simulink model "QD2_IOCheck_2021b"  (R2021b)
settings: Solver=ode2  StartTime=0.0  StopTime=inf  FixedStep=1/1000  RelTol=1e-3  EnableMultiTasking=on
InitFcn:
  | Motor_Mapping_7_Inch
undefined symbols (not defined in the file): datetime, HIL, KT, log_QD2_, m, Motor_Matrix, qc_get_step_size, saved_data
libraries: quarc_library x44, simulink x6, simulink_extras x1
(part 1 of 2)
settings Model: DataTypeOverride=Double  MinMaxOverflowLogging=ForceOff  SimulationMode=external  ExtModeTrigElement=1  ExtModeTrigDuration=10000  ExtModeTrigLevel=0.400000  Creator=dmadill  LastModifiedBy=jpineros
settings SolverCC: AlgebraicLoopSolver=TrustRegion  PositivePriorityOrder=on  AutoInsertRateTranBlk=on
settings DataIOCC: ReturnWorkspaceOutputs=off
settings DebuggingCC: ArithmeticOperatorsInVariantConditions=warning
settings HardwareCC: ProdBitPerLong=64  ProdLargestAtomicInteger=LongLong  ProdLargestAtomicFloat=Double  ProdLongLongMode=on  ProdHWDeviceType=ARM Compatible->ARM 64-bit (LP64)
settings SFSimCC: SimUseLocalCustomCode=off  CustomCodeUndefinedFunction=UseInterfaceOnly
settings RTWCC: Description=QUARC Linux QDrone2 Target Using Toolchain  SystemTargetFile=quarc_linux_qdrone2.tlc  RTWUseLocalCustomCode=off  Toolchain=QUARC linux_qdrone2 | gmake (64-bit Windows)  BuildConfiguration=Faster Runs
settings CodeAppCC: StateflowObjectComments=on
settings STFCustomTargetCC: ConcurrentExecutionCompliant=on  UseToolchainInfoCompliant=on  SystemTargetFile=quarc_linux_qdrone2.tlc
settings GRTTargetCC: TargetLangStandard=C89/C90 (ANSI)  ParMdlRefBuildCompliant=off  CompOptLevelCompliant=off  CombineOutputUpdateFcns=off  MatFileLogging=off  CPPClassGenCompliant=off  GRTInterface=on  ExtMode=on  ExtModeMexFile=quarc_comm  ExtModeMexArgs='-w -d /tmp -uri %u','tcpip://192.168.55.1:17001'
settings ConfigComp: CovMetricSettings=dswe

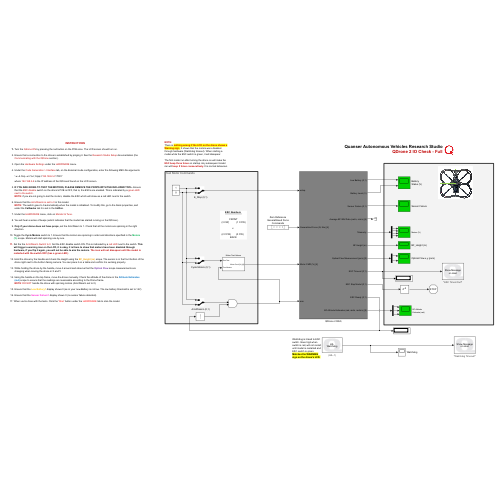
[thumbnail: Simulink's stored preview of the top-level diagram]
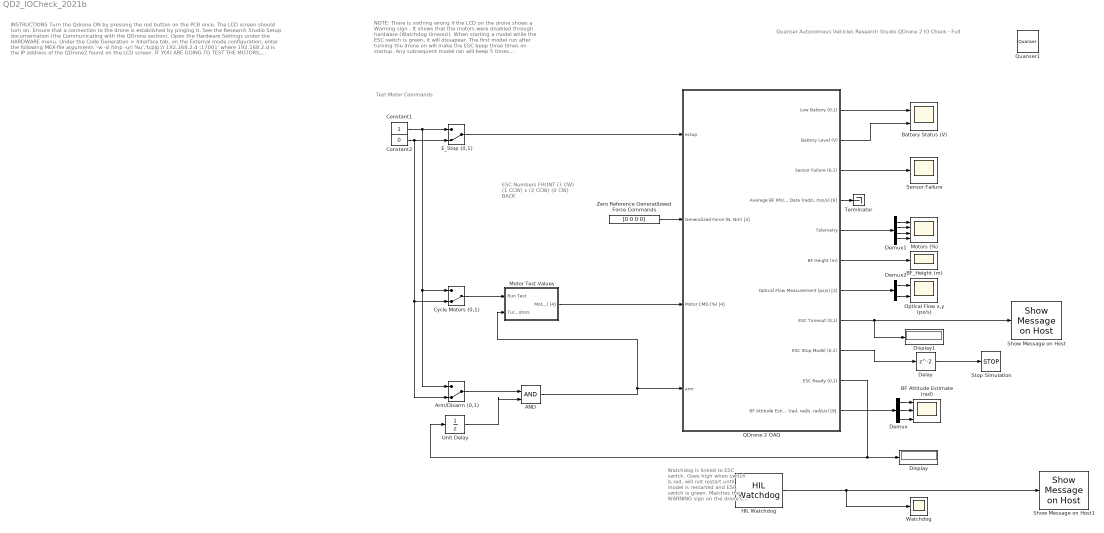
== system QD2_IOCheck_2021b ==
  note: Watchdog is linked to ESC switch. Goes high when switch is red, will not restart until model is restarted and ESC switch is green.
      | Matches the WARNING sign on the drone's LCD.
  note: Test Motor Commands
  note: Quanser Autonomous Vehicles Research Studio
      | QDrone 2 IO Check - Full
  note: ESC Numbers
      |
      | FRONT
      | (3 CW) (1 CCW)
      |
      | x
      |
      | (2 CCW) (0 CW)
      | BACK
  note: INSTRUCTIONS
      |
      | Turn the Qdrone ON by pressing the red button on the PCB once. The LCD screen should turn on.
      |
      | Ensure that a connection to the drone is established by pinging it. See the Research Studio Setup documentation (the Communicating with the QDrone section).
      |
      | Open the Hardware Settings under the HARDWARE menu.
      |
      | Under the Code Generation > Interface tab, on the External mode configuration, enter the following MEX-file arguments
      |
      | '-w -d /tmp -uri %u','tcpip:// 192.168.2.d :17001'
      |
      | where 192.168.2.d is the IP address of the QDrone2 found on the LCD screen.
      |
      | IF YOU ARE GOING TO TEST THE MOTORS, PLEASE REMOVE THE PROPS WITH THE INCLUDED TOOL. Ensure that the ESC disable switch on the drone's PCB is OFF, that is, the ESCs are enabled. This is indicated by a green LED next to the switch .
      | NOTE: if you are not going to test the motors, disable the ESC which will show as a red LED next to the switch.
      |
      | Ensure that the Arm/Disarm is set to 0 in this model.
      | NOTE: The switch goes to 0 automatically when the model is initialized. To modify this, go to the block properties, and under the Callbacks tab it is set in the InitFcn .
      |
      | Under the HARDWARE menu, click on Monitor & Tune .
      |
      | You will hear a series of beeps (which indicates that the model has started running on the QDrone).
      |
      | Only if your drone does not have props, set the Arm/Disarn to 1. Check that all the motors are spinning in the right direction.
      |
      | Toggle the Cycle Motors switch to 1. Ensure that the motors are spinning in order and directions specified in the Motors (%) scope. Motors will start spinning one by one.
      |
      | Set the the Arm/Disarm Switch to 0. Set the ESC disable switch ON. This is indicated by a red LED next to the switch. This will trigger a warning icon on the LCD, it is okay, it is there to show that motors have been disabled through hardware, if you flip it again, you will not be able to arm the motors. The icon will not dissapear until the model is restarted with the switch OFF (has a green LED.)
      |
      | Hold the drone by the handle and check the Height using the BF_Height (m) scope. The sensor is in the front bottom of the drone right next to the bottom facing camera. You can place it on a table and confirm it is working properly.
      |
      | While holding the drone by the handle, move it around and observe that the Optical Flow scope measurements are changing when moving the drone in X and Y.
      |
      | Using the handle on the top frame, move the drone manually. Check the attitude of the drone in the Attitude Estimates (rad) scope to ensure that the readings are reasonable according to the Drone frame.
      | NOTE : DO NOT handle the drone with spinning motors (Arm/Disarm set to 0).
      |
      | Ensure that the Low Battery? display shows 0 (as in your new Battery is not low. The low battery threshold is set to 14V)
      |
      | Ensure that the Sensor Failure? display shows 0 (no sensor failure detected).
      |
      | When you're done with the tests, Click the ' Stop ' button under the HARDWARE tab to stop the model.
  note: NOTE:
      | There is nothing wrong if the LCD on the drone shows a Warning sign . It shows that the motors were disabled through hardware (Watchdog timeout). When starting a model while the ESC switch is green, it will dissapear.
      |
      | The first model run after turning the drone on will make the ESC beep three times on startup. Any subsequent model ran will beep 5 times consecutively. It is normal behaviour.
  AND : Logic  IconShape=distinctive  AllPortsSameDT=off  OutDataTypeStr=boolean
  Arm/Disarm (0,1) : ManualSwitch  InitFcn=set_param(gcb,'sw','0')  CurrentSetting=0
  "BF Attitude Estimate (rad) " : Scope  NumInputPorts=3
  BF_Height (m) : Scope
  Battery Status (V) : Scope  NumInputPorts=2
  Constant1 : Constant
  Constant2 : Constant  Value=0
  Cycle Motors (0,1) : ManualSwitch  InitFcn=set_param(gcb,'sw','0')  CurrentSetting=0
  Delay : Delay
  Demux : Demux  Outputs=3
  Demux1 : Demux
  Demux2 : Demux  Outputs=2
  Display : Display
  Display1 : Display
  E_Stop (0,1) : ManualSwitch  CurrentSetting=0
  HIL Watchdog : quarc_library/Data Acquisition/Generic/Watchdog/HIL Watchdog  object_name=HIL-1  timeout=0.1  sample_time=qc_get_step_size  active=off
      settings: AttributesFormatString=(%<object_name>)  SourceProductName=QUARC Targets
  Motor Test Values : Subsystem
  Motors (%) : Scope  NumInputPorts=4
  Optical Flow x,y (px/s) : Scope  NumInputPorts=2
  QDrone 2 DAQ : Subsystem
  Quanser1 : quarc_library/Logos/Quanser
  Sensor Failure : Scope
  Show Message on Host : quarc_library/Sinks/Error Handling/Show Message on Host  message_type=Fixed error message  message_icon=Error  message=ESC Timed Out!
      settings: AttributesFormatString="\"%<message>\""  SourceProductName=QUARC Targets
  Show Message on Host1 : quarc_library/Sinks/Error Handling/Show Message on Host  message_type=Fixed error message  message_icon=Error  message=Watchdog Timeout!
      settings: AttributesFormatString="\"%<message>\""  SourceProductName=QUARC Targets
  Stop Simulation : Stop
  Terminator : Terminator
  Unit Delay : UnitDelay  SampleTime=-1  HasFrameUpgradeWarning=on
  Watchdog : Scope
  Zero Reference Generatlizeed Force Commands : Constant  Value=[0 0 0 0]
  wires:
  Constant2/1 -> Arm/Disarm (0,1)/2, Cycle Motors (0,1)/2, E_Stop (0,1)/2
  Constant1/1 -> E_Stop (0,1)/1, Arm/Disarm (0,1)/1, Cycle Motors (0,1)/1
  Demux/1 -> "BF Attitude Estimate (rad) "/1
  Demux/2 -> "BF Attitude Estimate (rad) "/2
  Demux/3 -> "BF Attitude Estimate (rad) "/3
  Demux2/1 -> Optical Flow x,y (px/s)/1
  Demux2/2 -> Optical Flow x,y (px/s)/2
  Demux1/3 -> Motors (%)/3
  Demux1/2 -> Motors (%)/2
  Demux1/4 -> Motors (%)/4
  Demux1/1 -> Motors (%)/1
  HIL Watchdog/1 -> Show Message on Host1/1, Watchdog/1
  Cycle Motors (0,1)/1 -> Motor Test Values/1(Run Test)
  E_Stop (0,1)/1 -> QDrone 2 DAQ/1(estop)
  Motor Test Values/1(Motor Cmd (%) [4]) -> QDrone 2 DAQ/3(Motor CMD (%) [4])
  QDrone 2 DAQ/5(Telemetry) -> Demux1/1
  QDrone 2 DAQ/1(Low Battery (0,1)) -> Battery Status (V)/1
  QDrone 2 DAQ/2(Battery Level (V)) -> Battery Status (V)/2
  QDrone 2 DAQ/6(BF Height (m)) -> BF_Height (m)/1
  QDrone 2 DAQ/7(Optical Flow Measurement (px/s) [2]) -> Demux2/1
  QDrone 2 DAQ/4("Average BF IMU Data (rad/s, m/s/s) [6]") -> Terminator/1
  QDrone 2 DAQ/3(Sensor Failure (0,1)) -> Sensor Failure/1
  QDrone 2 DAQ/10(ESC Ready (0,1)) -> Unit Delay/1, Display/1
  AND/1 -> QDrone 2 DAQ/4(arm), Motor Test Values/2(Turn Motors)
  Arm/Disarm (0,1)/1 -> AND/1
  Unit Delay/1 -> AND/2
  QDrone 2 DAQ/9(ESC Stop Model (0,1)) -> Delay/1
  QDrone 2 DAQ/8(ESC Timeout (0,1)) -> Show Message on Host/1, Display1/1
  Delay/1 -> Stop Simulation/1
  QDrone 2 DAQ/11("BF Attitude Estimates (rad, rad/s, rad/s/s) [9]") -> Demux/1
  Zero Reference Generatlizeed Force Commands/1 -> QDrone 2 DAQ/2("Generalized Force (N, Nm) [4]")

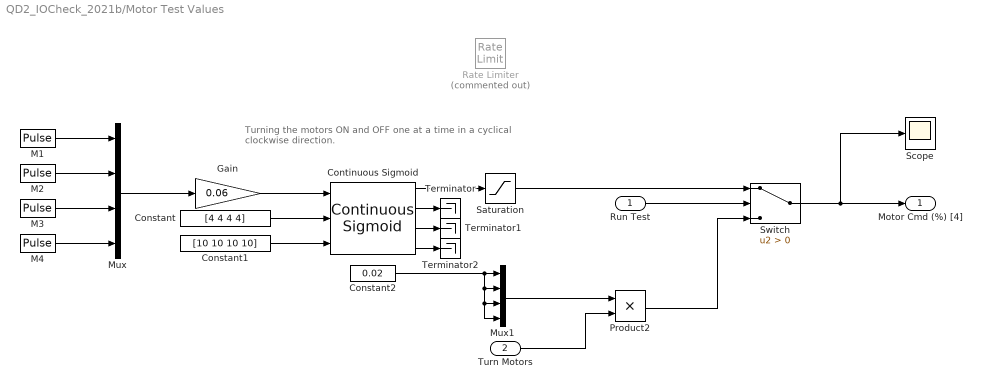
== system QD2_IOCheck_2021b/Motor Test Values ==
  note: Turning the motors ON and OFF one at a time in a cyclical
      | clockwise direction.
  Run Test : Inport
  Turn Motors : Inport  Port=2
  Constant : Constant  Value=[4 4 4 4]
  Constant1 : Constant  Value=[10 10 10 10]
  Constant2 : Constant  Value=0.02
  Continuous Sigmoid : quarc_library/Sources/Sigmoids/Continuous Sigmoid  params_source=External (input ports)  max_velocity=10  max_acceleration=10  initial_position=0  initial_velocity=0  hold_off=0.5  input_sample_time=-1  output_sample_time=qc_get_step_size
      settings: SourceProductName=QUARC Targets
  Gain : Gain  Gain=0.06
  M1 : DiscretePulseGenerator  PulseType=Time based  Period=8  PulseWidth=12.5
  M2 : DiscretePulseGenerator  PulseType=Time based  Period=8  PulseWidth=12.5  PhaseDelay=6
  M3 : DiscretePulseGenerator  PulseType=Time based  Period=8  PulseWidth=12.5  PhaseDelay=2
  M4 : DiscretePulseGenerator  PulseType=Time based  Period=8  PulseWidth=12.5  PhaseDelay=4
  Mux : Mux
  Mux1 : Mux
  Product2 : Product
  Rate Limiter : RateLimiter  Commented=on  RisingSlewLimit=0.1  FallingSlewLimit=-0.1  SampleTimeMode=inherited
  Saturation : Saturate  UpperLimit=0.1  LowerLimit=0.02
  Scope : Scope
  Switch : Switch  Criteria=u2 > Threshold
  Terminator : Terminator
  Terminator1 : Terminator
  Terminator2 : Terminator
  Motor Cmd (%) [4] : Outport  VectorParamsAs1DForOutWhenUnconnected=off
  wires:
  M2/1 -> Mux/2
  M3/1 -> Mux/3
  M4/1 -> Mux/4
  M1/1 -> Mux/1
  Continuous Sigmoid/1 -> Saturation/1
  Mux/1 -> Gain/1
  Gain/1 -> Continuous Sigmoid/1
  Constant/1 -> Continuous Sigmoid/2
  Constant1/1 -> Continuous Sigmoid/3
  Product2/1 -> Switch/3
  Saturation/1 -> Switch/1
  Turn Motors/1 -> Product2/2
  Switch/1 -> Motor Cmd (%) [4]/1, Scope/1
  Run Test/1 -> Switch/2
  Mux1/1 -> Product2/1
  Constant2/1 -> Mux1/2, Mux1/4, Mux1/3, Mux1/1
  Continuous Sigmoid/2 -> Terminator/1
  Continuous Sigmoid/3 -> Terminator1/1
  Continuous Sigmoid/4 -> Terminator2/1

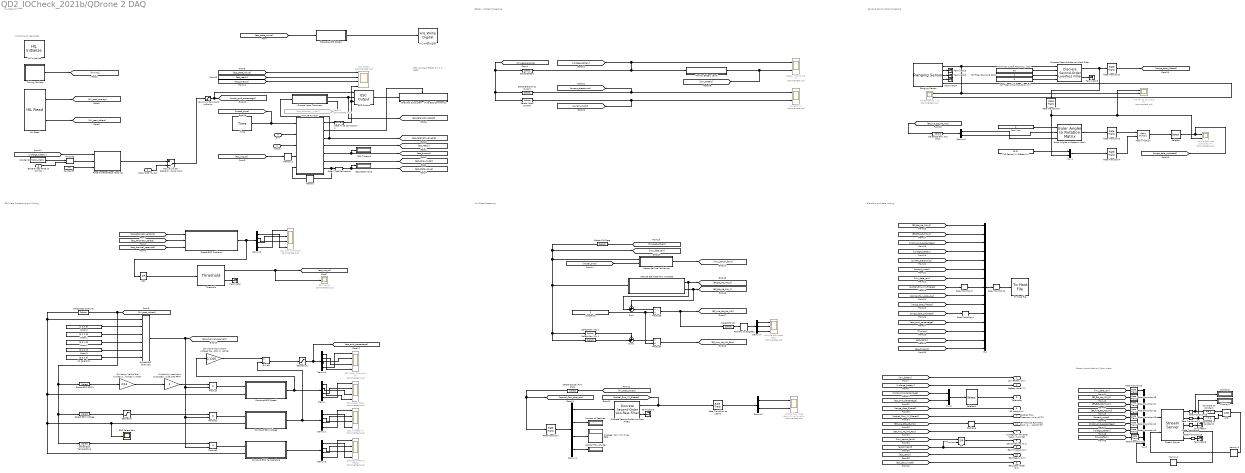
== system QD2_IOCheck_2021b/QDrone 2 DAQ ==
  note: Stream drone data to Python class
  note: HIL Read Write
  note: Blackbox and data routing
  note: ESC Numbers
      |
      | FRONT
      | 3 1
      |
      | 2 0
      | BACK
  note: Ranging Sensor Data Processing
  note: Initialize and read data
  note: ESC Data Processing and Writing
  note: IMU Data Processing
  note: Battery Voltage Processing
  estop : Inport
  "Generalized Force (N, Nm) [4]" : Inport  Port=2
  Motor CMD (%) [4] : Inport  Port=3
  arm : Inport  Port=4
  AND : Logic  IconShape=distinctive  AllPortsSameDT=off  OutDataTypeStr=boolean
  Attitude Estimate from IMU Data : Subsystem
  Attitude Estimates (deg) : Scope  Commented=on  NumInputPorts=3
  "Average, Max, Min Pixel Rate" : Display
  Battery Monitoring (V) : Scope  Commented=on  NumInputPorts=2
  Choose Motor Telemetry : Subsystem
  Compare To Constant : simulink/Logic and Bit Operations/Compare To Constant  relop===  const=2  OutDataTypeStr=boolean
  Compare To Constant1 : simulink/Logic and Bit Operations/Compare To Constant  relop=>=  const=0  OutDataTypeStr=boolean
  Constant1 : Constant  Value=2
  Constant2 : Constant  Value=Motor_Matrix  OutDataTypeStr=double
  Constant3 : Constant  Value=KT  OutDataTypeStr=double
  Construct ESC Speed : Subsystem
  Construct ESC Temperature : Subsystem
  Construct ESC Voltage : Subsystem
  Convert to equivalent voltage (based on motor Kv rating) : Gain  Gain=1/1300
  Currents (A) : Scope  Commented=on  NumInputPorts=2
  Data Type Conversion : DataTypeConversion  OutDataTypeStr=uint32
  Data Type Conversion1 : DataTypeConversion
  Demux{,1..3,8} (5 alike) : Demux
  Demux4 : Demux  Outputs=[2 1 3 1]
  Demux5 : Demux  Outputs=2
  Demux6 : Demux  Outputs=2
  Demux7 : Demux  Outputs=3
  Detect ESC Problems : Subsystem
  Discrete Second-Order Low-Pass Filter : quarc_library/Discrete/Discrete Second-Order Low-Pass Filter  params_source=External (input ports)  input_width=1  input_zeta=1  input_init=0  sample_time=qc_get_step_size*ceil(1/25/qc_get_step_size)
      settings: SourceProductName=QUARC Targets
  Discrete Second-Order Low-Pass Filter1 : quarc_library/Discrete/Discrete Second-Order Low-Pass Filter  params_source=Internal (dialog parameters)  input_width=1  input_zeta=1  input_init=0  sample_time=0.01
      settings: SourceProductName=QUARC Targets
  Display5 : Display
  Display6 : Display
  Divide : Product  Inputs=*/
  Divide by half of the number of poles in motor : Gain  Gain=2/14
  ESC Comm Problem : Scope  Commented=on  NumInputPorts=4
  ESC Motor Command (%) : Scope  Commented=on  NumInputPorts=4
  ESC Not OK : Scope  Commented=on
  ESC Output : quarc_library/Data Acquisition/Generic/Transformations/ESC Output  protocol=DShot (raw)
      settings: AttributesFormatString=%<protocol>  SourceProductName=QUARC Targets
  ESC Select Raw : Scope
  ESC Speed (RPM) : Scope  Commented=on  NumInputPorts=4
  ESC State Value : Display
  ESC States : Scope  Commented=on  NumInputPorts=4
  ESC Temperature (degC) : Scope  Commented=on  NumInputPorts=4
  ESC Timeout : Display
  ESC Voltage (V) : Scope  Commented=on  NumInputPorts=4
  Enabled Subsystem - Write ESC Commands : Subsystem  TreatAsAtomicUnit=on
  Euler Angles to Rotation Matrix : quarc_library/Math Operations/Matrices/Euler Angles to Rotation Matrix  menu_order=Relative Z-Y-X
      settings: SourceProductName=QUARC Targets
  Extract ESC Channels : MultiPortSwitch  DataPortOrder=Zero-based contiguous  Inputs=4  DataPortForDefault=Additional data port  zeroidx=on
  Force to percentage Mapping : MATLAB Function  TreatAsAtomicUnit=on
  Generate LED Pattern : Subsystem
  Goto19 : Goto  Commented=on  GotoTag=esc_telemetry_index
  HIL Initialize : quarc_library/Data Acquisition/Generic/Configuration/HIL Initialize  object_name=HIL-1  board_type=qdrone2  board_number=0  board_options=gyro0_fs=250;gyro0_rate=500;gyro0_bw=125;gyro0_ord=3;accel0_fs=16;accel0_rate=1000;accel0_bw=250;accel0_ord=3;temp0_bw=4000;gyro1_fs=250;gyro1_rate=500;gyro1_bw=125;gyro1_ord=3;accel1_fs=16;accel1_rate=1000;accel1_bw=400;accel1_ord=3;temp1_bw=4000;enc0_dir=0;enc1_dir=0;pwm03_dshot=1;opt_rate=121;  exclusive=off  active=on  hardware_clocks=[]  clock_modes=[]  initial_clock_frequencies=[]  set_clock_params_at_start=off  set_clock_params_at_switch_in=off  set_clock_frequencies_at_start=off  set_clock_frequencies_at_switch_in=off  analog_input_channels=[0:3]  analog_input_configurations=[]  analog_input_maximums=[3.3]  analog_input_minimums=[0]  set_analog_input_params_at_start=off  set_analog_input_params_at_switch_in=off  analog_output_channels=[]  analog_output_maximums=[]  analog_output_minimums=[]  initial_analog_outputs=[]  final_analog_outputs=[]  watchdog_analog_outputs=[]  set_analog_output_params_at_start=off  set_analog_output_params_at_switch_in=off  set_analog_outputs_at_start=off  set_analog_outputs_at_switch_in=off  set_analog_outputs_at_terminate=off  set_analog_outputs_at_switch_out=off  set_analog_outputs_on_watchdog=off  digital_input_channels=[0:5]  digital_output_channels=[6:11]  digital_output_configuration=[]  initial_digital_outputs=[0]  final_digital_outputs=[0]  watchdog_digital_outputs=[0 0 0 0 0 0]  set_digital_output_params_at_start=off  set_digital_output_params_at_switch_in=off  set_digital_outputs_at_start=on  set_digital_outputs_at_switch_in=off  set_digital_outputs_at_terminate=on  set_digital_outputs_at_switch_out=off  set_digital_outputs_on_watchdog=off  encoder_channels=[0:1]  quadrature=[4]  encoder_filter_frequency=100e6/1  initial_encoder_counts=[0]  set_encoder_params_at_start=on  set_encoder_params_at_switch_in=off  set_encoder_counts_at_start=on  set_encoder_counts_at_switch_in=off  pwm_channels=[0:5]  pwm_modes=[6 6 6 6 0]  pwm_frequency=[600000]  pwm_configuration=[0]  pwm_alignment=[0]  pwm_polarity=[1]  pwm_leading_deadband=[]  pwm_trailing_deadband=[]  initial_pwm_outputs=[0]  final_pwm_outputs=[0]  watchdog_pwm_outputs=[0]  set_pwm_params_at_start=on  set_pwm_params_at_switch_in=off  set_pwm_outputs_at_start=on  set_pwm_outputs_at_switch_in=off  set_pwm_outputs_at_terminate=on  set_pwm_outputs_at_switch_out=off  set_pwm_outputs_on_watchdog=on  other_output_channels=[]  initial_other_outputs=[]  final_other_outputs=[]  watchdog_other_outputs=[]  set_other_outputs_at_start=on  set_other_outputs_at_switch_in=off  set_other_outputs_at_terminate=on  set_other_outputs_at_switch_out=off  set_other_outputs_on_watchdog=off
  HIL Read : quarc_library/Data Acquisition/Generic/Immediate I//O/HIL Read  object_name=HIL-1  analog_channels=[3 1:2]  encoder_channels=[]  digital_channels=[]  other_channels=[3000:3002 4000:4002 3003:3005 4003:4005 17000:17006 17008:17009 17007 17010]  sample_time=qc_get_step_size  active=on  vector_output=on  data_type_mode=Inherit via back propagation  encoder_data_type=double  digital_data_type=boolean
  HIL Write Digital : quarc_library/Data Acquisition/Generic/Immediate I//O/HIL Write Digital  object_name=HIL-1  channels=[6:11]  sample_time=-1  active=off  vector_input=on
      settings: SourceProductName=QUARC Targets
  Height Estimate Compares (m) : Scope  Commented=on  NumInputPorts=2
  MATLAB Function : MATLAB Function  TreatAsAtomicUnit=on
  Manual Switch - Select Command Input : ManualSwitch  CurrentSetting=0
  Matrix Multiply : Product  Multiplication=Matrix(*)
  "Maximum Command Authority " : Saturate  UpperLimit=[1 1 1 1]  LowerLimit=[1 1 1 1]*0.025
  Memory : Memory
  Memory1 : Memory
  Memory2 : Memory  InheritSampleTime=on
  Memory3 : Memory  InheritSampleTime=on
  Monitor Battery Level : Subsystem
  Motor 0 : Constant  Value=[1 0 0 0]
  Motor 1 : Constant  Value=[0 1 0 0]
  Motor 2 : Constant  Value=[0 0 1 0]
  Motor 3 : Constant  Value=[0 0 0 1]
  Multiple by resolution (supposed to be 100 RPM) : Gain
  Mux : Mux  Inputs=15
  Mux1 : Mux  Inputs=2
  Mux2 : Mux  Inputs=2
  Mux3 : Mux  Inputs=9
  No selection : Constant  Value=[0 0 0 0]
  Number of Features : Display
  OR : Logic  Operator=OR  IconShape=distinctive  AllPortsSameDT=off  OutDataTypeStr=boolean
  OR1 : Logic  Operator=OR  Inputs=1  IconShape=distinctive  AllPortsSameDT=off  OutDataTypeStr=boolean
  Optical Flow Rate (Body Frame) (pixel/s) : Scope  Commented=on  NumInputPorts=2
  Optical Flow Shutter : Display
  Product : Product
  Product1 : Product
  Product2 : Product
  Product3 : Product  Inputs=*/
  Product4 : Product  Inputs=*/
  Product5 : Product  Multiplication=Matrix(*)
  Radians to Degrees : simulink_extras/Transformations/Radians to Degrees
  Ranging Sensor : quarc_library/Devices/Third-Party/Sensors/Ranging Sensor  sensor_type=VL53L1X Time-of-flight  uri=i2c-cpu://localhost:0?address='0x29',baud='400000',memsize='512'  ranging_distance=Long  timing_budget=0.033  measurement_period=0.040  output_mode=Fixed-size output  samples_per_revolution=1300  max_distance=0.050  max_angle=5  sample_time=qc_get_step_size*ceil(1/25/qc_get_step_size)  show_versions=off  active=on
      settings: SourceProductName=QUARC Targets
  Rate Transition : RateTransition  OutPortSampleTime=0.01
  Rate Transition to 100Hz : RateTransition  OutPortSampleTime=0.01
  Rate Transition{1..2,7..12,14..20} (15 alike) : RateTransition
  Rate Transition3 : RateTransition  OutPortSampleTime=qc_get_step_size*ceil(1/25/qc_get_step_size)
  Rate Transition4 : RateTransition  OutPortSampleTime=qc_get_step_size*ceil(1/25/qc_get_step_size)
  Rate Transition5 : RateTransition  OutPortSampleTime=qc_get_step_size*ceil(1/25/qc_get_step_size)
  Rate Transition6 : RateTransition  OutPortSampleTime=qc_get_step_size
  Reshape : Reshape
  Saturation : Saturate  UpperLimit=17  LowerLimit=10
  Saturation1 : Saturate  UpperLimit=1  LowerLimit=0
  Select Battery : Selector  InputPortWidth=3  IndexOptions=Index vector (dialog)  Indices=[1]  OutputSizes=1
  Select ESC Channel : Selector  InputPortWidth=23  IndexOptions=Index vector (dialog)  Indices=[22]  OutputSizes=1
  Select ESC RPPM : Selector  InputPortWidth=23  IndexOptions=Index vector (dialog)  Indices=[20]  OutputSizes=1
  Select ESC Temperature : Selector  InputPortWidth=23  IndexOptions=Index vector (dialog)  Indices=[23]  OutputSizes=1
  Select ESC Voltage : Selector  InputPortWidth=23  IndexOptions=Index vector (dialog)  Indices=[21]  OutputSizes=1
  Select Electronics Current : Selector  InputPortWidth=3  IndexOptions=Index vector (dialog)  Indices=[2]  OutputSizes=1
  Select Est Att : Selector  InputPortWidth=9  IndexOptions=Index vector (dialog)  Indices=[1:3]  OutputSizes=1
  Select Est Roll and Pitch : Selector  InputPortWidth=9  IndexOptions=Index vector (dialog)  Indices=[1:2]  OutputSizes=1
  Select IMU Data : Selector  InputPortWidth=23  IndexOptions=Index vector (dialog)  Indices=[1:12]  OutputSizes=1
  Select Motor Current : Selector  InputPortWidth=3  IndexOptions=Index vector (dialog)  Indices=[3]  OutputSizes=1
  Select Optical Flow Data : Selector  InputPortWidth=23  IndexOptions=Index vector (dialog)  Indices=[13:19]  OutputSizes=1
  Select Raw IMU 0 : Selector  InputPortWidth=12  IndexOptions=Index vector (dialog)  Indices=[1:6]  OutputSizes=1
  Select Raw IMU 1 : Selector  InputPortWidth=12  IndexOptions=Index vector (dialog)  Indices=[7:12]  OutputSizes=1
  Selector : Selector  InputPortWidth=3  IndexOptions=Index vector (dialog)  Indices=[3]  OutputSizes=1
  Selector1 : Selector  InputPortWidth=8  IndexOptions=Index vector (dialog)  Indices=[4,8,3,7,2,6,1,5]  OutputSizes=1
  Sensor Failure Monitoring : Subsystem
  Stream Server : quarc_library/Communications/Basic/Stream Server  uri_source=Specify via dialog (do not evaluate)  uri=tcpip://localhost:18491?nagle='off'  send_buffer_size=1460  receive_buffer_size=1460  byte_order=little endian (Intel - LSB first)  optimization=Minimum latency  send_options=Send most recent data  receive_options=Receive most recent data  default_value=0  sample_time=qc_get_step_size*2  active=on  implementation=Use blocking I/O in a separate thread  send_fifo_size=1000  receive_fifo_size=1000  send_priority=0  receive_priority=0  send_dimensions=off  receive_dimensions=off  max_dimensions=-1  data_type=Inherited via back propagation  type_expr=BusObject
      settings: AttributesFormatString="\"tcpip://localhost:18491?nagle='off'\""
  Sum : Sum  Inputs=++|
  Sum1 : Sum  Inputs=++|
  Terminator{,1..7} (8 alike) : Terminator
  Threshold : quarc_library/Discontinuities/Threshold  operator=~=  param_src=Specify via dialog  threshold=0  duration=qc_get_step_size*300
      settings: SourceProductName=QUARC Targets
  Time : quarc_library/Sources/Time/Time  time_source=Wall clock  sample_time=qc_get_step_size
  Timing Monitors : Subsystem
  To Host File : quarc_library/Sinks/To Host/To Host File  source=Specify via dialog (do not evaluate)  file_name=saved_data\%m\log_QD2_%{regexprep(regexprep(char(datetime),':','-'),' ','_')}.mat  variable_name=QD2_data  decimation=1  sample_time=-1  file_format=MAT-file v.4  options=No header or footer  append=off  final_file_name=saved_data\\QD2_IOCheck_2021b_\\log_QD2_2025-05-01_13-49-19.mat  bitrate=2000000
  ToF Filter Cutoff Frequency (rad) : Constant  Value=40
  ToF Filter Damping Ratio : Constant
  ToF Filter Initial Condition (m) : Constant  Value=0
  ToF Range Compare (m) : Scope  Commented=on  NumInputPorts=2
  ToF Range Raw (m) : Scope  Commented=on  NumInputPorts=2
  ToF Sensor XY Offsets (m) : Constant  Value=[0 0]
  Zero Yaw : Constant  Value=0
  Low Battery (0,1) : Outport
  Battery Level (V) : Outport  Port=2
  Sensor Failure (0,1) : Outport  Port=3
  "Average BF IMU Data (rad/s, m/s/s) [6]" : Outport  Port=4
  Telemetry : Outport  Port=5
  BF Height (m) : Outport  Port=6
  Optical Flow Measurement (px/s) [2] : Outport  Port=7
  ESC Timeout (0,1) : Outport  Port=8
  ESC Stop Model (0,1) : Outport  Port=9
  ESC Ready (0,1) : Outport  Port=10
  "BF Attitude Estimates (rad, rad/s, rad/s/s) [9]" : Outport  Port=11
  wires:
  Mux3/1 -> Stream Server/1
  Stream Server/5 -> Rate Transition18/1
  Rate Transition16/1 -> Compare To Constant/1, Display5/1
  Rate Transition18/1 -> Terminator6/1  "Connected (bool)"
  Rate Transition14/1 -> Compare To Constant1/1, Display6/1
  Stream Server/3 -> Rate Transition9/1
  [imu_data_raw] -> Rate Transition8/1
  [current_motor] -> Rate Transition20/1
  Rate Transition15/1 -> Mux3/2
  [motor_cmd_percentage] -> Rate Transition10/1
  Rate Transition8/1 -> Mux3/1
  [voltage_battery] -> Rate Transition12/1
  Compare To Constant/1 -> AND/1
  [low_battery] -> Rate Transition11/1
  [BF_Est_Att_IMU_1] -> Rate Transition17/1
  Memory2/1 -> Mux3/9
  Compare To Constant1/1 -> AND/2
  Stream Server/4 -> Memory2/1
  Stream Server/2 -> Rate Transition14/1
  Rate Transition19/1 -> Mux3/4
  Rate Transition20/1 -> Mux3/5
  AND/1 -> Memory3/1
  [BF_Est_Att_IMU_0] -> Rate Transition15/1
  [BF_Ave_Est_Att_IMU] -> Rate Transition19/1
  Rate Transition12/1 -> Mux3/7
  Rate Transition11/1 -> Mux3/8
  Rate Transition17/1 -> Mux3/3
  Stream Server/1 -> Rate Transition16/1
  Rate Transition10/1 -> Mux3/6
  Rate Transition9/1 -> Terminator7/1
  Memory3/1 -> Stream Server/2
  Rate Transition7/1 -> Mux/8
  Rate Transition6/1 -> To Host File/1
  OR/1 -> Sensor Failure (0,1)/1
  Product2/1 -> Construct ESC Temperature/1(ESC Data In [4])
  Demux8/1 -> ESC Comm Problem/4
  Select ESC RPPM/1 -> Divide by half of the number of poles in motor/1
  Demux3/3 -> ESC Temperature (degC)/2
  ESC Output/1 -> Enabled Subsystem - Write ESC Commands/1(DShot Raw [4])
  arm/1 -> MATLAB Function/2(arm)
  Demux2/4 -> ESC Motor Command (%)/1
  Demux3/4 -> ESC Temperature (degC)/1
  Demux1/4 -> ESC Voltage (V)/1
  Divide by half of the number of poles in motor/1 -> Multiple by resolution (supposed to be 100 RPM)/1
  Select Battery/1 -> [voltage_battery], Battery Monitoring (V)/1, Monitor Battery Level/1(Battery (V))
  Extract ESC Channels/1 -> [esc_channel_received], Product/2, Product1/2, Product2/2
  Time/1 -> [model_time], MATLAB Function/1(mdl_time)
  [range_data_projected] -> Rate Transition1/1
  Choose Motor Telemetry/1(Motor telemetry select) -> [esc_telemetry_select], ESC Output/2
  Rate Transition2/1 -> [range_data_filtered]
  MATLAB Function/7(state) -> Data Type Conversion/1, Memory/1
  Data Type Conversion1/1 -> ESC States/4, ESC Output/3
  Motor 2/1 -> Extract ESC Channels/4
  Construct ESC Speed/1(ESC Data Out [4]) -> Demux/1, Convert to equivalent voltage (based on motor Kv rating)/1
  Demux2/1 -> ESC Motor Command (%)/4
  Rate Transition1/1 -> Mux/11
  Multiple by resolution (supposed to be 100 RPM)/1 -> Product/1
  Select Electronics Current/1 -> [current_electronics], Currents (A)/1
  Select ESC Channel/1 -> Extract ESC Channels/1, Construct ESC Temperature/2(ESC Channel Select), ESC Select Raw/1, Construct ESC Voltage/2(ESC Channel Select), Construct ESC Speed/2(ESC Channel Select)
  MATLAB Function/1(cmd) -> Data Type Conversion1/1
  Product4/1 -> [BF_Ave_Att_IMU_Raw]
  Motor 3/1 -> Extract ESC Channels/5
  Select Est Roll and Pitch/1 -> Demux6/1
  Demux3/2 -> ESC Temperature (degC)/3
  Motor 0/1 -> Extract ESC Channels/2
  Timing Monitors/1(Timings) -> [Timing]
  [hil_read_others] -> Select ESC RPPM/1, Select ESC Temperature/1, Select ESC Voltage/1, Select ESC Channel/1
  MATLAB Function/3(tele_enable) -> [esc_telemetry_enable], Choose Motor Telemetry/1(enable telemetry)
  Choose Motor Telemetry/2(Motor telemetry index) -> Goto19/1
  Constant1/1 -> Product4/2, Product3/2
  [esc_not_ok] -> Memory1/1
  Demux/1 -> ESC Speed (RPM)/4
  Rate Transition3/1 -> Matrix Multiply/1
  Demux/2 -> ESC Speed (RPM)/3
  Mux/1 -> Rate Transition6/1
  Demux2/3 -> ESC Motor Command (%)/2
  Motor 1/1 -> Extract ESC Channels/3
  Demux/4 -> ESC Speed (RPM)/1
  Detect ESC Problems/1(ESC Comm Problem [4]) -> OR1/1, Demux8/1
  Demux/3 -> ESC Speed (RPM)/2
  Rate Transition/1 -> Demux4/1
  Attitude Estimate from IMU Data/1("BF Estimated Attitude for IMU0 (rad, rad/s, rad/2^2) [9]") -> Sum/2, [BF_Est_Att_IMU_0]
  Selector/1 -> [range_data_projected], Height Estimate Compares (m)/1
  Demux8/3 -> ESC Comm Problem/2
  Select Optical Flow Data/1 -> [optical_flow_data_raw], Rate Transition/1
  Saturation/1 -> Product1/1
  Demux5/1 -> Optical Flow Rate (Body Frame) (pixel/s)/1
  Demux1/3 -> ESC Voltage (V)/2
  Data Type Conversion/1 -> [esc_state_value], ESC State Value/1
  Zero Yaw/1 -> Euler Angles to Rotation Matrix/1
  "Maximum Command Authority "/1 -> [motor_cmd_percentage], ESC Output/1
  Rate Transition5/1 -> ToF Range Compare (m)/1, Height Estimate Compares (m)/2, Mux1/2
  [hil_read_others] -> Select IMU Data/1
  Product/1 -> Construct ESC Speed/1(ESC Data In [4])
  Attitude Estimate from IMU Data/2("BF Estimated Attitude for IMU1 (rad, rad/s, rad/2^2) [9]") -> Sum/1, [BF_Est_Att_IMU_1]
  MATLAB Function/5(esc_timeout) -> [esc_timeout], ESC Timeout/1
  ToF Filter Damping Ratio/1 -> Discrete Second-Order Low-Pass Filter/3
  Demux8/2 -> ESC Comm Problem/3
  [hil_read_analog] -> Select Electronics Current/1, Select Motor Current/1, Select Battery/1
  OR1/1 -> Threshold/1
  [esc_timeout] -> ESC States/3
  [BF_Est_Att_IMU_0] -> Mux/1
  No selection/1 -> Extract ESC Channels/6
  Select IMU Data/1 -> [imu_data_raw], Sensor Failure Monitoring/1(IMU Data [12]), Attitude Estimate from IMU Data/1(IMU Data [12]), Select Raw IMU 0/1, Select Raw IMU 1/1
  Ranging Sensor/3 -> Terminator3/1
  MATLAB Function/2(cmd_enable) -> Enabled Subsystem - Write ESC Commands/Enable
  Ranging Sensor/1 -> ToF Range Compare (m)/2, ToF Range Raw (m)/1, Discrete Second-Order Low-Pass Filter/1
  ToF Filter Initial Condition (m)/1 -> Discrete Second-Order Low-Pass Filter/4
  MATLAB Function/4(esc_ready) -> [esc_ready]
  [esc_timeout] -> Mux/15
  Threshold/1 -> ESC Not OK/1, [esc_not_ok]
  Construct ESC Temperature/1(ESC Data Out [4]) -> Demux3/1
  Demux1/1 -> ESC Voltage (V)/4
  Construct ESC Voltage/1(ESC Data Out [4]) -> Divide/2, Demux1/1
  Select Motor Current/1 -> [current_motor], Currents (A)/2
  MATLAB Function/6(stop_mdl) -> [esc_stop_model]
  Select ESC Temperature/1 -> Product2/1
  Euler Angles to Rotation Matrix/1 -> Rate Transition3/1
  Demux8/4 -> ESC Comm Problem/1
  [model_time] -> Sensor Failure Monitoring/2(Model Time)
  Demux1/2 -> ESC Voltage (V)/3
  [esc_telemetry_enable] -> Detect ESC Problems/1(ESC Telemetry Enabled)
  HIL Read/2 -> [hil_read_others]
  Product1/1 -> Construct ESC Voltage/1(ESC Data In [4])
  Memory/1 -> MATLAB Function/5(pre_state)
  HIL Read/1 -> [hil_read_analog]
  Demux4/3 -> "Average, Max, Min Pixel Rate"/1
  Memory1/1 -> MATLAB Function/4(esc_problem)
  Discrete Second-Order Low-Pass Filter/1 -> Rate Transition5/1, Rate Transition2/1
  Generate LED Pattern/1(LED Command) -> HIL Write Digital/1
  [esc_channel_received] -> Detect ESC Problems/3(ESC Channel Reported [4])
  Threshold/2 -> Terminator/1
  Sum1/1 -> Product4/1
  Demux7/3 -> Attitude Estimates (deg)/3
  Rate Transition4/1 -> Matrix Multiply/2
  estop/1 -> MATLAB Function/3(estop)
  Demux2/2 -> ESC Motor Command (%)/3
  Discrete Second-Order Low-Pass Filter1/2 -> Terminator1/1
  [hil_read_others] -> Select Optical Flow Data/1
  [esc_state_value] -> ESC States/1
  Demux5/2 -> Optical Flow Rate (Body Frame) (pixel/s)/2
  [imu_data_raw] -> Mux/7
  Demux4/1 -> Discrete Second-Order Low-Pass Filter1/1  "Optical Flow Pixel Rate (XY)"
  Sum/1 -> Product3/1
  Product3/1 -> Select Est Att/1, [BF_Ave_Est_Att_IMU]
  Mux1/1 -> Rate Transition4/1
  Rate Transition to 100Hz/1 -> Demux5/1
  Demux4/2 -> Number of Features/1
  Convert to equivalent voltage (based on motor Kv rating)/1 -> Divide/1
  Demux3/1 -> ESC Temperature (degC)/4
  Monitor Battery Level/1(Low Battery) -> [low_battery], Battery Monitoring (V)/2
  Demux4/4 -> Optical Flow Shutter/1
  [motor_cmd_percentage] -> Mux/3
  Select ESC Voltage/1 -> Saturation/1
  Divide/1 -> Saturation1/1
  [esc_ready] -> ESC States/2
  [esc_telemetry_select] -> Detect ESC Problems/2(ESC Channel Request [4])
  [optical_flow_data_raw] -> Mux/9
  Select Raw IMU 1/1 -> Sum1/2
  Select Raw IMU 0/1 -> Sum1/1
  Matrix Multiply/1 -> Selector/1
  Select Est Att/1 -> Radians to Degrees/1
  [esc_state_value] -> Generate LED Pattern/1(ESC States)
  Sensor Failure Monitoring/1(Sensor Fault) -> [imu_sensor_fault]
  Demux7/2 -> Attitude Estimates (deg)/2
  Discrete Second-Order Low-Pass Filter1/1 -> [optical_flow_XY_filtered], Rate Transition to 100Hz/1
  [current_motor] -> Mux/6
  [Timing] -> Mux/13
  ToF Sensor XY Offsets (m)/1 -> Mux1/1
  ToF Filter Cutoff Frequency (rad)/1 -> Discrete Second-Order Low-Pass Filter/2
  Ranging Sensor/2 -> Terminator2/1
  Ranging Sensor/4 -> Terminator4/1
  Demux6/2 -> Euler Angles to Rotation Matrix/2
  Radians to Degrees/1 -> Demux7/1
  Discrete Second-Order Low-Pass Filter/2 -> Terminator5/1
  Ranging Sensor/5 -> ToF Range Raw (m)/2
  Demux7/1 -> Attitude Estimates (deg)/1
  Demux6/1 -> Euler Angles to Rotation Matrix/3
  [range_data_filtered] -> Mux/10
  [esc_ready] -> Mux/14
  [BF_Ave_Est_Att_IMU] -> Select Est Roll and Pitch/1
  [esc_cmd_percentage] -> Mux/12
  [optical_flow_XY_filtered] -> Rate Transition7/1
  [current_electronics] -> Mux/5
  [voltage_battery] -> Mux/4
  [BF_Est_Att_IMU_1] -> Mux/2
  [low_battery] -> Low Battery (0,1)/1
  [voltage_battery] -> Battery Level (V)/1
  [esc_cmd_percentage] -> Mux2/2
  [motor_cmd_percentage] -> Mux2/1
  Mux2/1 -> Selector1/1
  Selector1/1 -> Telemetry/1
  [range_data_filtered] -> BF Height (m)/1
  [optical_flow_XY_filtered] -> Optical Flow Measurement (px/s) [2]/1
  [BF_Ave_Est_Att_IMU] -> Reshape/1
  [imu_sensor_fault] -> OR/1
  [BF_Ave_Att_IMU_Raw] -> "Average BF IMU Data (rad/s, m/s/s) [6]"/1
  [esc_timeout] -> OR/2, ESC Timeout (0,1)/1
  [esc_ready] -> ESC Ready (0,1)/1
  [esc_stop_model] -> ESC Stop Model (0,1)/1
  Saturation1/1 -> [esc_cmd_percentage], Demux2/1
  Reshape/1 -> "BF Attitude Estimates (rad, rad/s, rad/s/s) [9]"/1
  Product5/1 -> Force to percentage Mapping/2(Motor_Forces)
  Constant3/1 -> Force to percentage Mapping/3(KT)
  Manual Switch - Select Command Input/1 -> "Maximum Command Authority "/1
  Constant2/1 -> Product5/1
  [voltage_battery] -> Force to percentage Mapping/1(V_Bat_Act)
  "Generalized Force (N, Nm) [4]"/1 -> Product5/2
  Motor CMD (%) [4]/1 -> Manual Switch - Select Command Input/2
  Force to percentage Mapping/1(Duty_Cycle) -> Manual Switch - Select Command Input/1

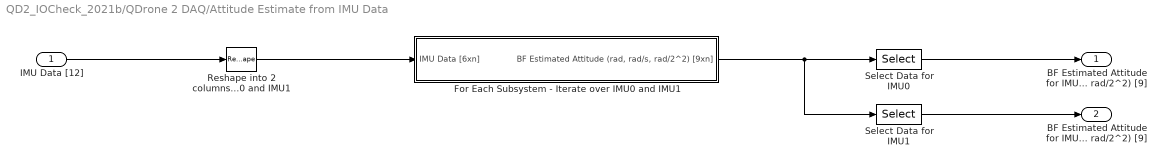
== system QD2_IOCheck_2021b/QDrone 2 DAQ/Attitude Estimate from IMU Data ==
  IMU Data [12] : Inport
  For Each Subsystem - Iterate over IMU0 and IMU1 : Subsystem  TreatAsAtomicUnit=on
  Reshape into 2 columns for IMU0 and IMU1 : Reshape  OutputDimensionality=Customize  OutputDimensions=[6,2]
  Select Data for IMU0 : Selector  NumberOfDimensions=2  InputPortWidth=3  IndexOptions=Index vector (dialog),Index vector (dialog)  Indices=[1:9],[1]  OutputSizes=1,1
  Select Data for IMU1 : Selector  NumberOfDimensions=2  InputPortWidth=3  IndexOptions=Index vector (dialog),Index vector (dialog)  Indices=[1:9],[2]  OutputSizes=1,1
  "BF Estimated Attitude for IMU0 (rad, rad/s, rad/2^2) [9]" : Outport
  "BF Estimated Attitude for IMU1 (rad, rad/s, rad/2^2) [9]" : Outport  Port=2
  wires:
  IMU Data [12]/1 -> Reshape into 2 columns for IMU0 and IMU1/1
  Reshape into 2 columns for IMU0 and IMU1/1 -> For Each Subsystem - Iterate over IMU0 and IMU1/1(IMU Data [6xn])
  For Each Subsystem - Iterate over IMU0 and IMU1/1("BF Estimated Attitude (rad, rad/s, rad/2^2) [9xn]") -> Select Data for IMU1/1, Select Data for IMU0/1
  Select Data for IMU0/1 -> "BF Estimated Attitude for IMU0 (rad, rad/s, rad/2^2) [9]"/1
  Select Data for IMU1/1 -> "BF Estimated Attitude for IMU1 (rad, rad/s, rad/2^2) [9]"/1

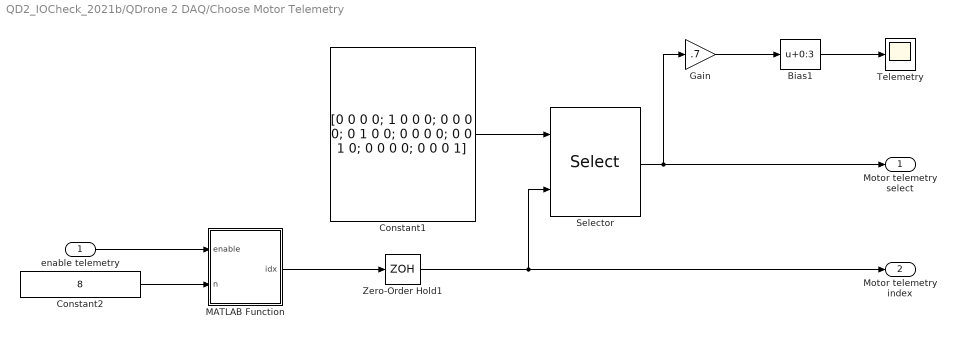
== system QD2_IOCheck_2021b/QDrone 2 DAQ/Choose Motor Telemetry ==
  enable telemetry : Inport
  Bias1 : Bias  Bias=0:3
  Constant1 : Constant  Value="[0 0 0 0; 1 0 0 0; 0 0 0 0; 0 1 0 0; 0 0 0 0; 0 0 1 0; 0 0 0 0;  0 0 0 1]"
  Constant2 : Constant  Value=8
  Gain : Gain  Gain=.7
  MATLAB Function : MATLAB Function  TreatAsAtomicUnit=on
  Selector : Selector  NumberOfDimensions=2  IndexMode=Zero-based  InputPortWidth=3  IndexOptions=Index vector (port),Select all  Indices=[1 3],1  OutputSizes=1,1
  Telemetry : Scope
  Zero-Order Hold1 : ZeroOrderHold  SampleTime=-1
  Motor telemetry select : Outport
  Motor telemetry index : Outport  Port=2
  wires:
  Gain/1 -> Bias1/1
  Bias1/1 -> Telemetry/1
  MATLAB Function/1(idx) -> Zero-Order Hold1/1
  Zero-Order Hold1/1 -> Selector/2, Motor telemetry index/1
  enable telemetry/1 -> MATLAB Function/1(enable)
  Selector/1 -> Motor telemetry select/1, Gain/1
  Constant1/1 -> Selector/1
  Constant2/1 -> MATLAB Function/2(n)

== system QD2_IOCheck_2021b/QDrone 2 DAQ/Construct ESC Speed ==
  ESC Data In [4] : Inport
  ESC Channel Select : Inport  Port=2
  For Each Subsystem - Construct ESC Signal : Subsystem  TreatAsAtomicUnit=on
  Memory : Memory  InitialCondition=zeros(1,4)
  ESC Data Out [4] : Outport
  wires:
  For Each Subsystem - Construct ESC Signal/1(ESC Data Out [4]) -> ESC Data Out [4]/1, Memory/1
  Memory/1 -> For Each Subsystem - Construct ESC Signal/3(ESC Previous Data [4])
  ESC Data In [4]/1 -> For Each Subsystem - Construct ESC Signal/1(ESC Data In [4])
  ESC Channel Select/1 -> For Each Subsystem - Construct ESC Signal/2(ESC Channel)

== system QD2_IOCheck_2021b/QDrone 2 DAQ/Construct ESC Temperature ==
  ESC Data In [4] : Inport
  ESC Channel Select : Inport  Port=2
  For Each Subsystem - Construct ESC Signal : Subsystem  TreatAsAtomicUnit=on
  Memory : Memory  InitialCondition=zeros(1,4)
  ESC Data Out [4] : Outport
  wires:
  For Each Subsystem - Construct ESC Signal/1(ESC Data Out [4]) -> ESC Data Out [4]/1, Memory/1
  Memory/1 -> For Each Subsystem - Construct ESC Signal/3(ESC Previous Data [4])
  ESC Data In [4]/1 -> For Each Subsystem - Construct ESC Signal/1(ESC Data In [4])
  ESC Channel Select/1 -> For Each Subsystem - Construct ESC Signal/2(ESC Channel)

== system QD2_IOCheck_2021b/QDrone 2 DAQ/Construct ESC Voltage ==
  ESC Data In [4] : Inport
  ESC Channel Select : Inport  Port=2
  For Each Subsystem - Construct ESC Signal : Subsystem  TreatAsAtomicUnit=on
  Memory : Memory  InitialCondition=zeros(1,4)
  ESC Data Out [4] : Outport
  wires:
  ESC Channel Select/1 -> For Each Subsystem - Construct ESC Signal/2(ESC Channel)
  ESC Data In [4]/1 -> For Each Subsystem - Construct ESC Signal/1(ESC Data In [4])
  Memory/1 -> For Each Subsystem - Construct ESC Signal/3(ESC Previous Data [4])
  For Each Subsystem - Construct ESC Signal/1(ESC Data Out [4]) -> Memory/1, ESC Data Out [4]/1

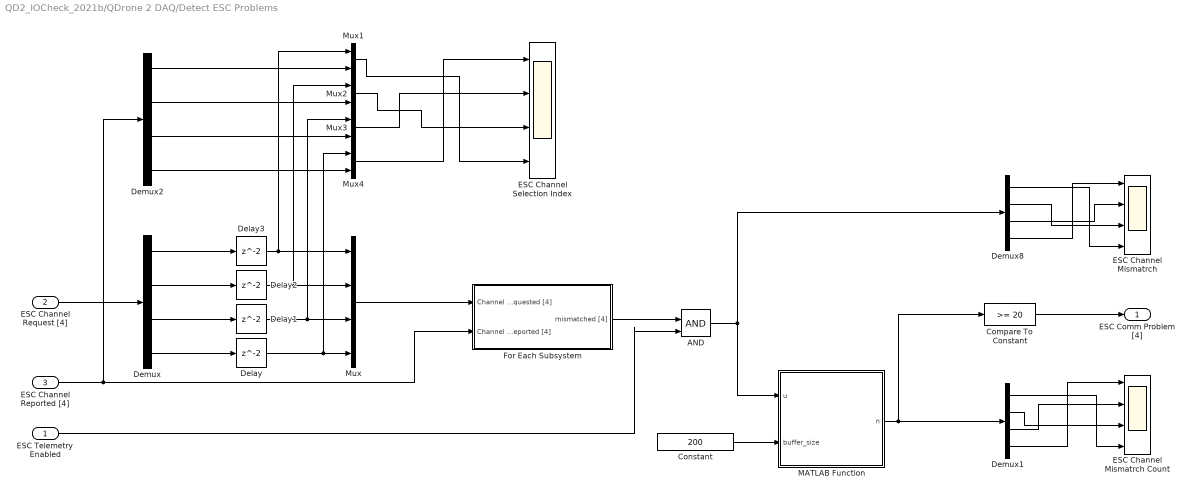
== system QD2_IOCheck_2021b/QDrone 2 DAQ/Detect ESC Problems ==
  ESC Telemetry Enabled : Inport
  ESC Channel Request [4] : Inport  Port=2
  ESC Channel Reported [4] : Inport  Port=3
  AND : Logic  IconShape=distinctive  AllPortsSameDT=off  OutDataTypeStr=boolean
  Compare To Constant : simulink/Logic and Bit Operations/Compare To Constant  relop=>=  const=20  OutDataTypeStr=boolean
  Constant : Constant  Value=200
  Delay{,1..3} (4 alike) : Delay
  Demux{,1..2,8} (4 alike) : Demux
  ESC Channel Mismatrch : Scope  NumInputPorts=4
  ESC Channel Mismatrch Count : Scope  NumInputPorts=4
  ESC Channel Selection Index : Scope  NumInputPorts=4
  For Each Subsystem : Subsystem  TreatAsAtomicUnit=on
  MATLAB Function : MATLAB Function  TreatAsAtomicUnit=on
  Mux : Mux
  Mux{1..4} (4 alike) : Mux  Inputs=2
  ESC Comm Problem [4] : Outport
  wires:
  ESC Channel Reported [4]/1 -> Demux2/1, For Each Subsystem/2(Channel Reported [4])
  Demux/1 -> Delay3/1
  Demux/2 -> Delay2/1
  Demux/3 -> Delay1/1
  Demux/4 -> Delay/1
  ESC Channel Request [4]/1 -> Demux/1
  Delay2/1 -> Mux2/1, Mux/2
  Delay3/1 -> Mux/1, Mux1/1
  Delay1/1 -> Mux3/1, Mux/3
  Delay/1 -> Mux4/1, Mux/4
  Mux/1 -> For Each Subsystem/1(Channel Requested [4])
  For Each Subsystem/1(mismatched [4]) -> AND/1
  AND/1 -> MATLAB Function/1(u), Demux8/1
  Demux8/2 -> ESC Channel Mismatrch/3
  Demux8/1 -> ESC Channel Mismatrch/4
  Demux8/3 -> ESC Channel Mismatrch/2
  Demux8/4 -> ESC Channel Mismatrch/1
  Constant/1 -> MATLAB Function/2(buffer_size)
  Demux1/4 -> ESC Channel Mismatrch Count/1
  Demux1/3 -> ESC Channel Mismatrch Count/2
  Demux1/1 -> ESC Channel Mismatrch Count/4
  Demux1/2 -> ESC Channel Mismatrch Count/3
  MATLAB Function/1(n) -> Compare To Constant/1, Demux1/1
  Compare To Constant/1 -> ESC Comm Problem [4]/1
  ESC Telemetry Enabled/1 -> AND/2
  Demux2/1 -> Mux1/2
  Demux2/2 -> Mux2/2
  Demux2/3 -> Mux3/2
  Demux2/4 -> Mux4/2
  Mux4/1 -> ESC Channel Selection Index/1
  Mux3/1 -> ESC Channel Selection Index/2
  Mux2/1 -> ESC Channel Selection Index/3
  Mux1/1 -> ESC Channel Selection Index/4

== system QD2_IOCheck_2021b/QDrone 2 DAQ/Enabled Subsystem - Write ESC Commands ==
  DShot Raw [4] : Inport
  Enable : EnablePort
  HIL Write PWM : quarc_library/Data Acquisition/Generic/Immediate I//O/HIL Write PWM  object_name=HIL-1  channels=[0:3]  sample_time=-1  active=off  vector_input=on
      settings: AttributesFormatString=(%<object_name>)  SourceProductName=QUARC Targets
  wires:
  DShot Raw [4]/1 -> HIL Write PWM/1

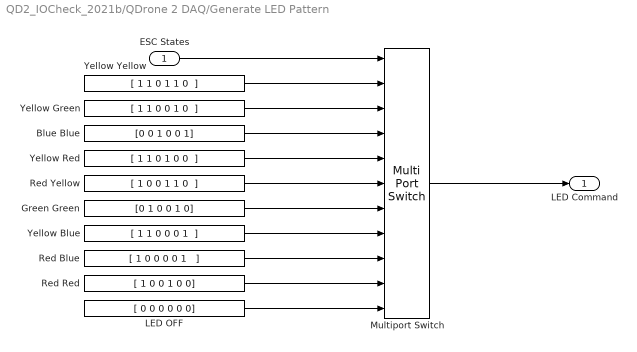
== system QD2_IOCheck_2021b/QDrone 2 DAQ/Generate LED Pattern ==
  ESC States : Inport
  Blue Blue : Constant  Value=[0 0 1 0 0 1]
  Green Green : Constant  Value=[0 1 0 0 1 0]
  LED OFF : Constant  Value=[ 0 0 0 0 0 0]
  Multiport Switch : MultiPortSwitch  DataPortOrder=Specify indices  DataPortIndices={0,1,2,3,4,5,77,88,99}  DataPortForDefault=Additional data port  DiagnosticForDefault=Warning
  Red Blue : Constant  Value="[ 1 0 0 0 0 1   ]"
  Red Red : Constant  Value=[ 1 0 0 1 0 0]
  Red Yellow : Constant  Value="[ 1 0 0 1 1 0  ]"
  Yellow Blue : Constant  Value="[ 1 1 0 0 0 1  ]"
  Yellow Green : Constant  Value="[ 1 1 0 0 1 0  ]"
  Yellow Red : Constant  Value="[ 1 1 0 1 0 0  ]"
  Yellow Yellow : Constant  Value="[ 1 1 0 1 1 0  ]"
  LED Command : Outport
  wires:
  Multiport Switch/1 -> LED Command/1
  ESC States/1 -> Multiport Switch/1
  Blue Blue/1 -> Multiport Switch/4
  Red Red/1 -> Multiport Switch/10
  Yellow Yellow/1 -> Multiport Switch/2
  Red Blue/1 -> Multiport Switch/9
  Yellow Blue/1 -> Multiport Switch/8
  LED OFF/1 -> Multiport Switch/11
  Green Green/1 -> Multiport Switch/7
  Yellow Green/1 -> Multiport Switch/3
  Yellow Red/1 -> Multiport Switch/5
  Red Yellow/1 -> Multiport Switch/6

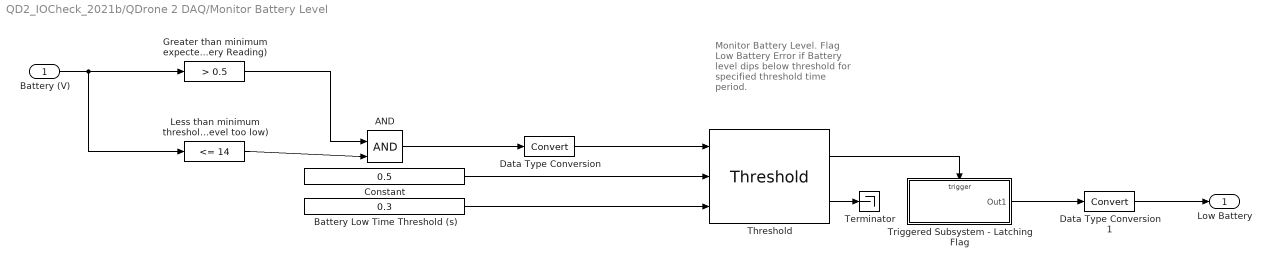
== system QD2_IOCheck_2021b/QDrone 2 DAQ/Monitor Battery Level ==
  note: Monitor Battery Level.
      | Flag Low Battery Error if
      | Battery level dips below
      | threshold for specified
      | threshold time period.
  Battery (V) : Inport
  AND : Logic  IconShape=distinctive  AllPortsSameDT=off  OutDataTypeStr=boolean
  Battery Low Time Threshold (s) : Constant  Value=0.3
  Constant : Constant  Value=0.5
  Data Type Conversion : DataTypeConversion
  Data Type Conversion1 : DataTypeConversion
  Greater than minimum expected voltage (Valid Battery Reading) : simulink/Logic and Bit Operations/Compare To Constant  relop=>  const=0.5  OutDataTypeStr=boolean
  Less than minimum threshold voltage (Battery level too low) : simulink/Logic and Bit Operations/Compare To Constant  relop=<=  const=14  OutDataTypeStr=boolean
  Terminator : Terminator
  Threshold : quarc_library/Discontinuities/Threshold  operator=>=  param_src=External input port  threshold=0  duration=0
      settings: SourceProductName=QUARC Targets
  Triggered Subsystem - Latching Flag : Subsystem  TreatAsAtomicUnit=on
  Low Battery : Outport
  wires:
  Battery (V)/1 -> Less than minimum threshold voltage (Battery level too low)/1, Greater than minimum expected voltage (Valid Battery Reading)/1
  Less than minimum threshold voltage (Battery level too low)/1 -> AND/2
  Greater than minimum expected voltage (Valid Battery Reading)/1 -> AND/1
  AND/1 -> Data Type Conversion/1
  Constant/1 -> Threshold/2
  Battery Low Time Threshold (s)/1 -> Threshold/3
  Data Type Conversion/1 -> Threshold/1
  Threshold/2 -> Terminator/1
  Threshold/1 -> Triggered Subsystem - Latching Flag/Trigger
  Triggered Subsystem - Latching Flag/1(Out1) -> Data Type Conversion1/1
  Data Type Conversion1/1 -> Low Battery/1

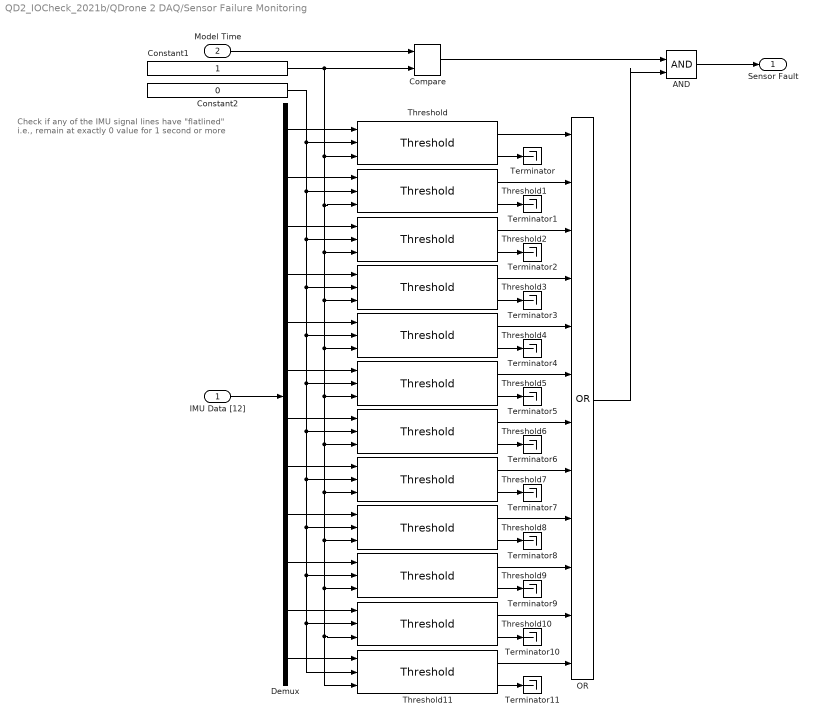
== system QD2_IOCheck_2021b/QDrone 2 DAQ/Sensor Failure Monitoring ==
  note: Check if any of the IMU signal lines have "flatlined"
      | i.e., remain at exactly 0 value for 1 second or more
  IMU Data [12] : Inport
  Model Time : Inport  Port=2
  AND : Logic  IconShape=distinctive  AllPortsSameDT=off  OutDataTypeStr=boolean
  Compare : quarc_library/Logic Operations/Compare  operator=>=  output_data_type=boolean
      settings: SourceProductName=QUARC Targets
  Constant1 : Constant
  Constant2 : Constant  Value=0
  Demux : Demux  Outputs=12
  OR : Logic  Operator=OR  Inputs=12  AllPortsSameDT=off  OutDataTypeStr=boolean
  Terminator{,1..11} (12 alike) : Terminator
  Threshold{,1..11} (12 alike) : quarc_library/Discontinuities/Threshold  operator===  param_src=External input port  threshold=0  duration=1
      settings: SourceProductName=QUARC Targets
  Sensor Fault : Outport
  wires:
  Model Time/1 -> Compare/1
  Constant1/1 -> Threshold1/3, Threshold2/3, Threshold3/3, Threshold5/3, Threshold6/3, Threshold7/3, Threshold8/3, Threshold9/3, Threshold10/3, Threshold11/3, Threshold4/3, Threshold/3, Compare/2
  Demux/1 -> Threshold/1
  Demux/2 -> Threshold1/1
  Constant2/1 -> Threshold1/2, Threshold2/2, Threshold3/2, Threshold4/2, Threshold5/2, Threshold6/2, Threshold7/2, Threshold8/2, Threshold9/2, Threshold10/2, Threshold11/2, Threshold/2
  IMU Data [12]/1 -> Demux/1
  Demux/3 -> Threshold2/1
  Demux/4 -> Threshold3/1
  Demux/5 -> Threshold4/1
  Demux/6 -> Threshold5/1
  Demux/7 -> Threshold6/1
  Demux/8 -> Threshold7/1
  Demux/9 -> Threshold8/1
  Demux/10 -> Threshold9/1
  Demux/11 -> Threshold10/1
  Demux/12 -> Threshold11/1
  Threshold/1 -> OR/1
  Threshold1/1 -> OR/2
  Threshold2/1 -> OR/3
  Threshold3/1 -> OR/4
  Threshold4/1 -> OR/5
  Threshold5/1 -> OR/6
  Threshold6/1 -> OR/7
  Threshold7/1 -> OR/8
  Threshold8/1 -> OR/9
  Threshold9/1 -> OR/10
  Threshold10/1 -> OR/11
  Threshold11/1 -> OR/12
  Threshold/2 -> Terminator/1
  Threshold1/2 -> Terminator1/1
  Threshold2/2 -> Terminator2/1
  Threshold3/2 -> Terminator3/1
  Threshold4/2 -> Terminator4/1
  Threshold5/2 -> Terminator5/1
  Threshold6/2 -> Terminator6/1
  Threshold7/2 -> Terminator7/1
  Threshold8/2 -> Terminator8/1
  Threshold9/2 -> Terminator9/1
  Threshold10/2 -> Terminator10/1
  Threshold11/2 -> Terminator11/1
  Compare/1 -> AND/1
  OR/1 -> AND/2
  AND/1 -> Sensor Fault/1

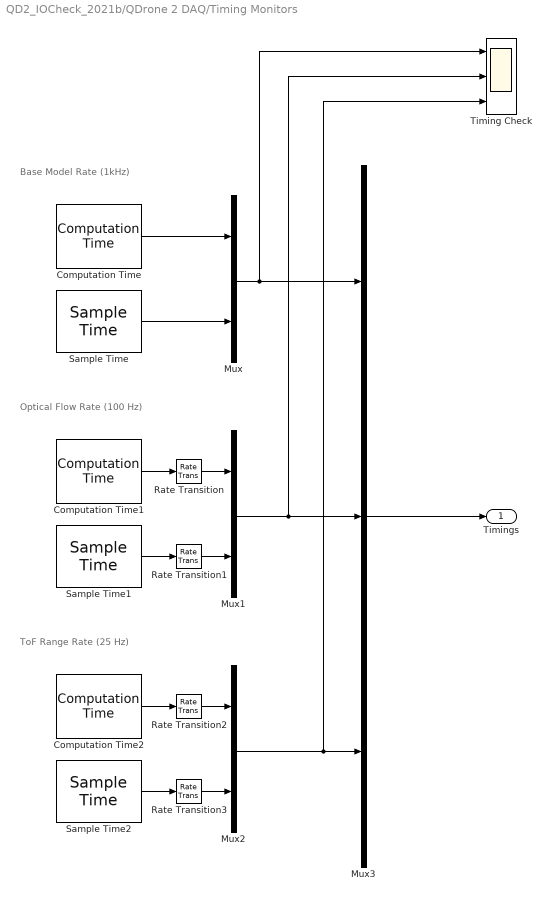
== system QD2_IOCheck_2021b/QDrone 2 DAQ/Timing Monitors ==
  note: Base Model Rate (1kHz)
  note: Optical Flow Rate (100 Hz)
  note: ToF Range Rate (25 Hz)
  Computation Time : quarc_library/Sources/Time/Computation Time  sample_time=qc_get_step_size  use_model=on  use_cpu_time=off
  Computation Time1 : quarc_library/Sources/Time/Computation Time  sample_time=0.01  use_model=on  use_cpu_time=off
  Computation Time2 : quarc_library/Sources/Time/Computation Time  sample_time=0.04  use_model=on  use_cpu_time=off
  Mux : Mux  Inputs=2
  Mux1 : Mux  Inputs=2
  Mux2 : Mux  Inputs=2
  Mux3 : Mux  Inputs=3
  Rate Transition{,1..3} (4 alike) : RateTransition
  Sample Time : quarc_library/Sources/Time/Sample Time  Priority=-99  sample_time=qc_get_step_size
  Sample Time1 : quarc_library/Sources/Time/Sample Time  Priority=-99  sample_time=0.01
  Sample Time2 : quarc_library/Sources/Time/Sample Time  Priority=-99  sample_time=0.04
  Timing Check : Scope  NumInputPorts=3
  Timings : Outport
  wires:
  Computation Time/1 -> Mux/1
  Sample Time/1 -> Mux/2
  Sample Time1/1 -> Rate Transition1/1
  Computation Time1/1 -> Rate Transition/1
  Computation Time2/1 -> Rate Transition2/1
  Sample Time2/1 -> Rate Transition3/1
  Mux1/1 -> Mux3/2, Timing Check/2
  Mux/1 -> Timing Check/1, Mux3/1
  Mux2/1 -> Timing Check/3, Mux3/3
  Mux3/1 -> Timings/1
  Rate Transition/1 -> Mux1/1
  Rate Transition1/1 -> Mux1/2
  Rate Transition2/1 -> Mux2/1
  Rate Transition3/1 -> Mux2/2
